simulink model "H_Sim_SingleGflInfiniteBus"  (R2020b)
settings: Solver=FixedStepAuto  StartTime=0  StopTime=4  FixedStep=Ts  RelTol=1e-3
undefined symbols (not defined in the file or in its folder): DeviceDiscreDamping, DevicePara, DevicePowerFlow, DeviceType, OtherInputs, PowerFlow, Ts, Wbase, x_e, Ybase, Zbase
libraries: SimplexPS x7, powerlib x7
settings Model: Creator=admin_user  LastModifiedBy=admin_user
settings DataIOCC: ReturnWorkspaceOutputs=off

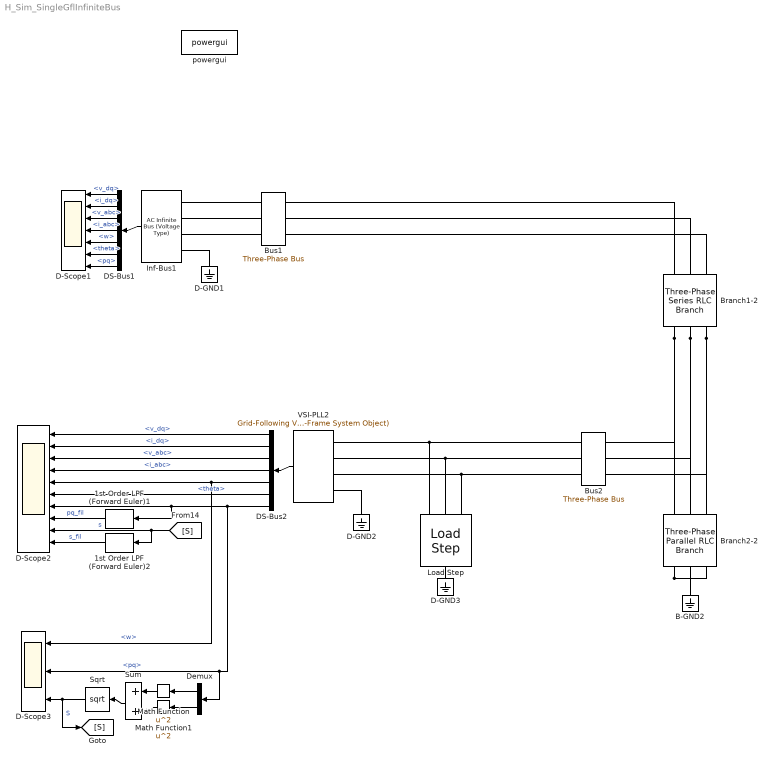
== system H_Sim_SingleGflInfiniteBus ==
  1st Order LPF (Forward Euler)1 : SimplexPS/1st Order LPF (Forward Euler)  wc=2*pi*100  Ts=Ts
      settings: SourceProductName=Simplex Power Systems
  1st Order LPF (Forward Euler)2 : SimplexPS/1st Order LPF (Forward Euler)  wc=2*pi*100  Ts=Ts
      settings: SourceProductName=Simplex Power Systems
  B-GND2 : powerlib/Elements/Ground  LConnTagsString=a
  Branch1-2 : powerlib/Elements/Three-Phase Series RLC Branch  LConnTagsString=A|B|C  RConnTagsString=A|B|C  BranchType=RL  Resistance=(0.03)*Zbase  Inductance=(0.3)*Zbase/Wbase  Capacitance=1e-6  Measurements=None
  Branch2-2 : powerlib/Elements/Three-Phase Parallel RLC Branch  LConnTagsString=A|B|C  RConnTagsString=A|B|C  BranchType=C  Resistance=(Inf)*Zbase  Inductance=1e-3  Capacitance=(0.01)*Ybase/Wbase  Measurements=None
      settings: SourceProductBaseCode=PS
  Bus1 : SimplexPS/Three-Phase Bus  Vbase=1  Sbase=1
      settings: SourceProductName=Simplex Power Systems
  Bus2 : SimplexPS/Three-Phase Bus  Vbase=1  Sbase=1
      settings: SourceProductName=Simplex Power Systems
  D-GND1 : powerlib/Elements/Ground  LConnTagsString=a
  D-GND2 : powerlib/Elements/Ground  LConnTagsString=a
  D-GND3 : powerlib/Elements/Ground  LConnTagsString=a
  D-Scope1 : Scope  NumInputPorts=7
  D-Scope2 : Scope  NumInputPorts=10
  D-Scope3 : Scope  NumInputPorts=3
  DS-Bus1 : BusSelector  OutputSignals=v_dq,i_dq,v_abc,i_abc,w,theta,pq
  DS-Bus2 : BusSelector  OutputSignals=v_dq,i_dq,v_abc,i_abc,w,theta,pq
  Demux : Demux  Outputs=2
  Inf-Bus1 : SimplexPS/AC Infinite Bus (Voltage Type)  Ts=Ts  Sbase=Sbase  Vbase=Vbase  Wbase=Wbase  vd=PowerFlow{1}(3)  vq=0  theta0=PowerFlow{1}(4)  w=Wbase  R=1e-30
      settings: SourceProductName=Simplex Power Systems
  Load Step : SimplexPS/Load Step  t0=2  R=2*Zbase  Reverse=0
      settings: SourceProductName=Simplex Power Systems
  Math Function : Math  Operator=square  SaturateOnIntegerOverflow=on
  Math Function1 : Math  Operator=square  SaturateOnIntegerOverflow=on
  Sqrt : Sqrt  SaturateOnIntegerOverflow=on
  Sum : Sum
  VSI-PLL2 : SimplexPS/Grid-Following Voltage-Source Inverter (dq-Frame System Object)  Ts=Ts  Sbase=Sbase  Vbase=Vbase  Wbase=Wbase  DeviceType=DeviceType{2}  DevicePara=DevicePara{2}  PowerFlow=DevicePowerFlow{2}  x0=x_e{2}  OtherInputs=OtherInputs{2}  DiscreMethod=Hybrid Trapezoidal  EnableInsideModification=off  DiscreDampingFlag=on  DiscreDampingValue=DeviceDiscreDamping{2}  LinearizationTimes=1  DirectFeedthrough=off
      settings: SourceProductName=Simplex Power Systems
  powergui : powerlib/powergui  Priority=1  SimulationMode=Discrete  SampleTime=Ts  frequency=60  Iterations=50  frequencyindice=0  Pbase=100e6  ErrMax=1e-4  UnitsV=kV  UnitsW=MW  buscounter=0  FunctionMessages=off  echomessages=off  EnableUseOfTLC=off  CurrentSourceSwitches=off  DisableSnubberDevices=off  DisableRonSwitches=off  DisableVfSwitches=off  DisplayEquations=off  AutomaticDiscreteSolvers=off  SolverType=Tustin/Backward Euler (TBE)  Interpol=off  ExternalGateDelay=off  methode=off  Ts=100  x0status=blocks  SPID=on  SwTol=0  HookPort=off  NonlinearTolerance=1e-4  nMaxIteration=100  ContinueOnMaxIteration=off  RestoreLinks=warning  ResistiveCurrentMeasurement=off  Frange=[0:2:500]  Ylog=off  Xlog=on  ShowGrid=off  save=off  variable=ZData  structure=0  ZoomFFT=off  StartTime=0.0  cycles=1  DisplayStyle=1  fundamental=60  FreqAxis=off  MaxFrequency=1000  frequencyindicesteady=1  RmsSteady=1  display=off
  wires:
  Inf-Bus1/1 -> DS-Bus1/1
  DS-Bus1/1 -> D-Scope1/1  "<v_dq>"
  DS-Bus1/2 -> D-Scope1/2  "<i_dq>"
  DS-Bus1/3 -> D-Scope1/3  "<v_abc>"
  DS-Bus1/4 -> D-Scope1/4  "<i_abc>"
  DS-Bus1/5 -> D-Scope1/5  "<w>"
  DS-Bus1/6 -> D-Scope1/6  "<theta>"
  DS-Bus1/7 -> D-Scope1/7  "<pq>"
  VSI-PLL2/1 -> DS-Bus2/1
  DS-Bus2/1 -> D-Scope2/1  "<v_dq>"
  DS-Bus2/2 -> D-Scope2/2  "<i_dq>"
  DS-Bus2/3 -> D-Scope2/3  "<v_abc>"
  DS-Bus2/4 -> D-Scope2/4  "<i_abc>"
  DS-Bus2/5 -> D-Scope3/1, D-Scope2/5  "<w>"
  DS-Bus2/6 -> D-Scope2/6  "<theta>"
  DS-Bus2/7 -> 1st Order LPF (Forward Euler)1/1, D-Scope2/7, Demux/1, D-Scope3/2  "<pq>"
  Demux/1 -> Math Function/1
  Demux/2 -> Math Function1/1
  Math Function/1 -> Sum/1
  Math Function1/1 -> Sum/2
  Sum/1 -> Sqrt/1
  Sqrt/1 -> [S], D-Scope3/3  "S"
  1st Order LPF (Forward Euler)1/1 -> D-Scope2/8  "pq_fil"
  [S] -> 1st Order LPF (Forward Euler)2/1, D-Scope2/9  "s"
  1st Order LPF (Forward Euler)2/1 -> D-Scope2/10  "s_fil"
  connections:
  Inf-Bus1/LConn4 -- D-GND1/LConn1
  VSI-PLL2/LConn4 -- D-GND2/LConn1
  Branch2-2/RConn1 -- Branch2-2/RConn2 -- Branch2-2/RConn3 -- B-GND2/LConn1
  Branch1-2/RConn1 -- Bus2/RConn1 -- Branch2-2/LConn1
  Branch1-2/RConn2 -- Bus2/RConn2 -- Branch2-2/LConn2
  Branch1-2/RConn3 -- Bus2/RConn3 -- Branch2-2/LConn3
  Bus1/RConn1 -- Branch1-2/LConn1
  Bus1/RConn2 -- Branch1-2/LConn2
  Bus1/RConn3 -- Branch1-2/LConn3
  Inf-Bus1/LConn1 -- Bus1/LConn1
  Inf-Bus1/LConn2 -- Bus1/LConn2
  Inf-Bus1/LConn3 -- Bus1/LConn3
  VSI-PLL2/LConn1 -- Load Step/LConn1 -- Bus2/LConn1
  VSI-PLL2/LConn2 -- Load Step/LConn2 -- Bus2/LConn2
  VSI-PLL2/LConn3 -- Load Step/LConn3 -- Bus2/LConn3
  D-GND3/LConn1 -- Load Step/RConn1
